simulink model "utils"  (Simulink 7.7)
settings: Solver=ode45  StartTime=0.0  StopTime=10.0  RelTol=1e-3
libraries: simulink x1, dspsigops x1
settings Model: Creator=iron  LastModifiedBy=iron

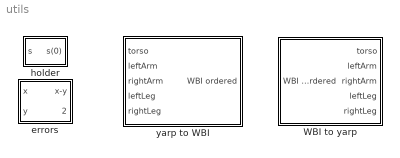
== system utils ==
  WBI to yarp : Subsystem
  errors : Subsystem
  holder : Subsystem
  yarp to WBI : Subsystem

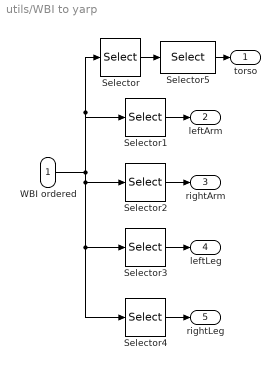
== system utils/WBI to yarp ==
  WBI ordered : Inport
  Selector : Selector  InputPortWidth=25  IndexOptions=Index vector (dialog)  Indices=[1 2 3]  OutputSizes=1
  Selector1 : Selector  InputPortWidth=25  IndexOptions=Index vector (dialog)  Indices=[4 5 6 7 8]  OutputSizes=1
  Selector2 : Selector  InputPortWidth=25  IndexOptions=Index vector (dialog)  Indices=[9 10 11 12 13]  OutputSizes=1
  Selector3 : Selector  InputPortWidth=25  IndexOptions=Index vector (dialog)  Indices=[14 15 16 17 18 19]  OutputSizes=1
  Selector4 : Selector  InputPortWidth=25  IndexOptions=Index vector (dialog)  Indices=[20 21 22 23 24 25]  OutputSizes=1
  Selector5 : Selector  InputPortWidth=3  IndexOptions=Index vector (dialog)  Indices=[3 2 1]  OutputSizes=1
  torso : Outport
  leftArm : Outport  Port=2
  rightArm : Outport  Port=3
  leftLeg : Outport  Port=4
  rightLeg : Outport  Port=5
  wires:
  Selector5/1 -> torso/1
  Selector/1 -> Selector5/1
  WBI ordered/1 -> Selector3/1, Selector4/1, Selector2/1, Selector1/1, Selector/1
  Selector4/1 -> rightLeg/1
  Selector3/1 -> leftLeg/1
  Selector2/1 -> rightArm/1
  Selector1/1 -> leftArm/1

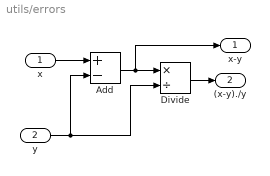
== system utils/errors ==
  x : Inport
  y : Inport  Port=2
  Add : Sum  Inputs=+-
  Divide : Product  Inputs=*/
  x-y : Outport
  (x-y)./y : Outport  Port=2
  wires:
  Divide/1 -> (x-y)./y/1
  y/1 -> Divide/2, Add/2
  x/1 -> Add/1
  Add/1 -> x-y/1, Divide/1

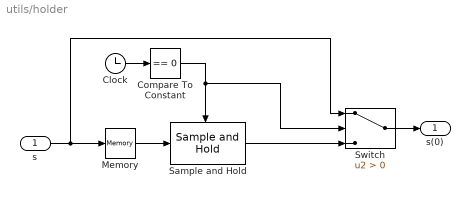
== system utils/holder ==
  s : Inport
  Clock : Clock
      settings: Decimation=10
  Compare To Constant : simulink/Logic and Bit Operations/Compare To Constant  SystemSampleTime=-1  relop===  const=0  LogicOutDataTypeMode=boolean
  Memory : Memory
  Sample and Hold : dspsigops/Sample and Hold  SystemSampleTime=-1  trig=Falling edge  initCond=0  latchinput=off
  Switch : Switch  Criteria=u2 > Threshold
  s(0) : Outport
  wires:
  Memory/1 -> Sample and Hold/1
  Switch/1 -> s(0)/1
  Sample and Hold/1 -> Switch/3
  Compare To Constant/1 -> Switch/2, Sample and Hold/Trigger
  Clock/1 -> Compare To Constant/1
  s/1 -> Memory/1, Switch/1

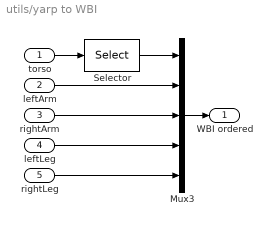
== system utils/yarp to WBI ==
  torso : Inport
  leftArm : Inport  Port=2
  rightArm : Inport  Port=3
  leftLeg : Inport  Port=4
  rightLeg : Inport  Port=5
  Mux3 : Mux  Inputs=5
  Selector : Selector  InputPortWidth=3  IndexOptions=Index vector (dialog)  Indices=[3 2 1]  OutputSizes=1
  WBI ordered : Outport
  wires:
  rightLeg/1 -> Mux3/5
  leftLeg/1 -> Mux3/4
  Mux3/1 -> WBI ordered/1
  rightArm/1 -> Mux3/3
  leftArm/1 -> Mux3/2
  torso/1 -> Selector/1
  Selector/1 -> Mux3/1
